simulink model "SimulationSimConnect"  (R2020b)
settings: Solver=FixedStepDiscrete  StartTime=0.0  StopTime=inf  RelTol=1e-3
InitFcn:
  | run('fbw_data_init_fbw_input.m')
values from neighbouring files (symbols this model uses):
  fbw_input_MATLABStruct = struct    [fbw_data_init_fbw_input.m]
undefined symbols (not defined in the file or in its folder): data, input, time
libraries: SimConnectToolbox x4, fbw_library x1, aerolibanimutils x1
settings Model: DataDictionary=fbw_data.sldd  Creator=Andreas  LastModifiedBy=Andreas
settings DebuggingCC: InheritedTsInSrcMsg=none

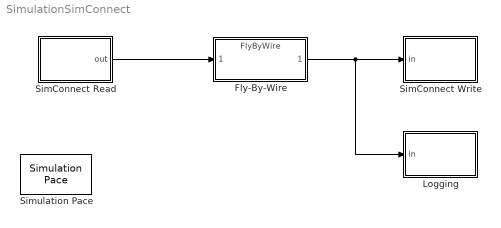
== system SimulationSimConnect ==
  Fly-By-Wire : ModelReference  ModelNameDialog=FlyByWire  ModelReferenceVersion=1.523
  Logging : Subsystem
  SimConnect Read : Subsystem
  SimConnect Write : Subsystem
  Simulation Pace : aerolibanimutils/Simulation Pace  SimulationPace=1  SleepMode=Auto  OutputPaceError=off  SampleTime=1/50
      settings: AttributesFormatString=%<SampleTime>
  wires:
  SimConnect Read/1(out) -> Fly-By-Wire/1
  Fly-By-Wire/1 -> Logging/1(in), SimConnect Write/1(in)

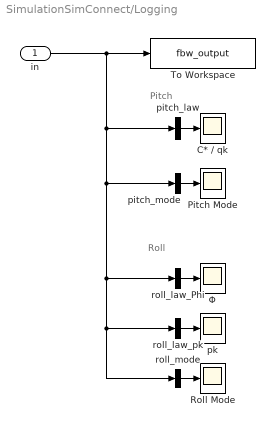
== system SimulationSimConnect/Logging ==
  note: Pitch
  note: Roll
  in : Inport
  C* / qk : Scope
  Pitch Mode : Scope
  Roll Mode : Scope
  To Workspace : ToWorkspace  VariableName=fbw_output  SaveFormat=Timeseries  SampleTime=-1
      settings: MaxDataPoints=30000
  pitch_law : BusSelector  OutputSignals=pitch.law_normal.nz_c_g,pitch.law_normal.Cstar_g,sim.data.nz_g,sim.data.qk_deg_s  OutputAsBus=on
  pitch_mode : BusSelector  OutputSignals=sim.data_computed.on_ground,pitch.data_computed.in_flight,pitch.data_computed.in_flare,pitch.data_computed.in_flight_gain  OutputAsBus=on
  pk : Scope
  roll_law_Phi : BusSelector  OutputSignals=roll.law_normal.Phi_c_deg,sim.data.Phi_deg  OutputAsBus=on
  roll_law_pk : BusSelector  OutputSignals=roll.law_normal.pk_c_deg_s,sim.data.pk_deg_s  OutputAsBus=on
  roll_mode : BusSelector  OutputSignals=sim.data_computed.on_ground,roll.data_computed.in_flight,roll.data_computed.in_flight_gain  OutputAsBus=on
  Φ : Scope
  wires:
  pitch_law/1 -> C* / qk/1
  roll_law_pk/1 -> pk/1
  roll_law_Phi/1 -> Φ/1
  in/1 -> To Workspace/1, pitch_law/1, roll_law_pk/1, roll_mode/1, roll_law_Phi/1, pitch_mode/1
  pitch_mode/1 -> Pitch Mode/1
  roll_mode/1 -> Roll Mode/1

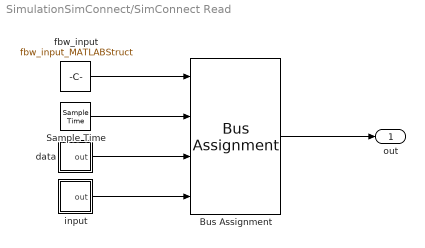
== system SimulationSimConnect/SimConnect Read ==
  Bus Assignment : BusAssignment  AssignedSignals=time.dt,data,input
  Sample Time : fbw_library/Sample Time  SystemSampleTime=-1  VariantActivationTime=update diagram  Latency=0  AutoFrameSizeCalculation=off
  data : Subsystem
  fbw_input : Constant  Value=fbw_input_MATLABStruct  OutDataTypeStr=Bus: fbw_input
  input : Subsystem
  out : Outport
  wires:
  fbw_input/1 -> Bus Assignment/1
  data/1(out) -> Bus Assignment/3
  Bus Assignment/1 -> out/1
  input/1(out) -> Bus Assignment/4
  Sample Time/1 -> Bus Assignment/2

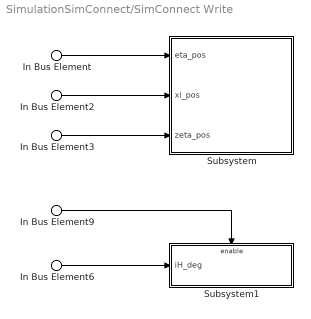
== system SimulationSimConnect/SimConnect Write ==
  In Bus Element : Inport  PortName=in  Element=sim.raw.output.eta_pos
  In Bus Element6 : Inport  PortName=in  Element=sim.raw.output.eta_trim_deg
  In Bus Element2 : Inport  PortName=in  Element=sim.raw.output.xi_pos
  In Bus Element3 : Inport  PortName=in  Element=sim.raw.output.zeta_pos
  In Bus Element9 : Inport  PortName=in  Element=sim.raw.output.eta_trim_deg_should_write
  Subsystem : Subsystem
  Subsystem1 : Subsystem
  wires:
  In Bus Element/1 -> Subsystem/1(eta_pos)
  In Bus Element2/1 -> Subsystem/2(xi_pos)
  In Bus Element3/1 -> Subsystem/3(zeta_pos)
  In Bus Element6/1 -> Subsystem1/1(iH_deg)
  In Bus Element9/1 -> Subsystem1/Enable

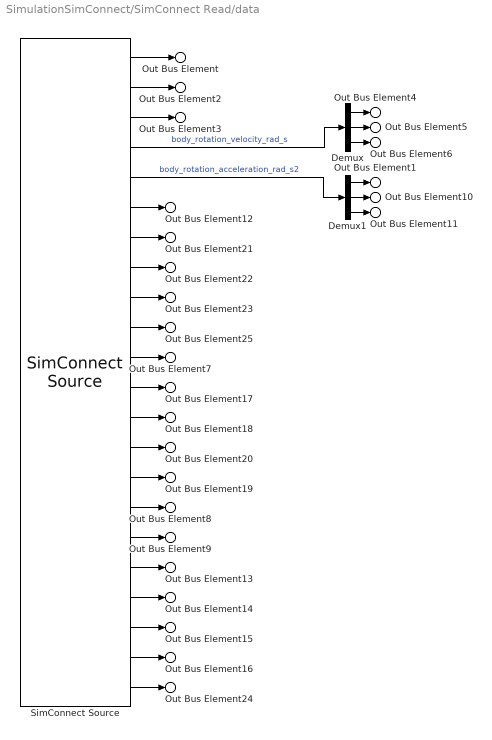
== system SimulationSimConnect/SimConnect Read/data ==
  Demux : Demux  Outputs=3
  Demux1 : Demux  Outputs=3
  SimConnect Source : SimConnectToolbox/SimConnect Source  configurationIndex=0  connectionName=SimConnectSource  variables=|
      | G FORCE, GFORCE;
      | PLANE PITCH DEGREES, DEGREE;
      | PLANE BANK DEGREES, DEGREE;
      | STRUCT BODY ROTATION VELOCITY, STRUCT;
      | STRUCT BODY ROTATION ACCELERATION, STRUCT;
      | ELEVATOR TRIM POSITION, DEGREE;
      | RUDDER TRIM PCT, PERCENT OVER 100;
      | INCIDENCE ALPHA, DEGREE;
      | INCIDENCE BETA, DEGREE;
      | BETA DOT, DEGREE PER SECOND;
      | AIRSPEED INDICATED, KNOTS;
      | AIRSPEED TRUE, KNOTS;
      | AIRSPEED MACH, MACH;
      | PLANE ALTITUDE, FEET;
      | INDICATED ALTITUDE, FEET;
      | RADIO HEIGHT, FEET;
      | CG PERCENT, PERCENT OVER 100;
      | GEAR ANIMATION POSITION:0, NUMBER;
      | GEAR ANIMATION POSITION:1, NUMBER;
      | GEAR ANIMATION POSITION:2, NUMBER;
      | FLAPS HANDLE INDEX, NUMBER;
      | AUTOPILOT MASTER, BOOL;
      settings: SourceProductName=SimConnect Toolbox
  Out Bus Element : Outport  PortName=out  Element=nz_g
  Out Bus Element2 : Outport  PortName=out  Element=Theta_deg
  Out Bus Element3 : Outport  PortName=out  Element=Phi_deg
  Out Bus Element4 : Outport  PortName=out  Element=q_rad_s
  Out Bus Element5 : Outport  PortName=out  Element=r_rad_s
  Out Bus Element6 : Outport  PortName=out  Element=p_rad_s
  Out Bus Element1 : Outport  PortName=out  Element=q_dot_rad_s2
  Out Bus Element10 : Outport  PortName=out  Element=r_dot_rad_s2
  Out Bus Element11 : Outport  PortName=out  Element=p_dot_rad_s2
  Out Bus Element12 : Outport  PortName=out  Element=eta_trim_deg
  Out Bus Element21 : Outport  PortName=out  Element=zeta_trim_pos
  Out Bus Element22 : Outport  PortName=out  Element=alpha_deg
  Out Bus Element23 : Outport  PortName=out  Element=beta_deg
  Out Bus Element25 : Outport  PortName=out  Element=beta_dot_deg_s
  Out Bus Element7 : Outport  PortName=out  Element=V_ias_kn
  Out Bus Element17 : Outport  PortName=out  Element=V_tas_kn
  Out Bus Element18 : Outport  PortName=out  Element=V_mach
  Out Bus Element20 : Outport  PortName=out  Element=H_ft
  Out Bus Element19 : Outport  PortName=out  Element=H_ind_ft
  Out Bus Element8 : Outport  PortName=out  Element=H_radio_ft
  Out Bus Element9 : Outport  PortName=out  Element=CG_percent_MAC
  Out Bus Element13 : Outport  PortName=out  Element=gear_animation_pos_0
  Out Bus Element14 : Outport  PortName=out  Element=gear_animation_pos_1
  Out Bus Element15 : Outport  PortName=out  Element=gear_animation_pos_2
  Out Bus Element16 : Outport  PortName=out  Element=flaps_handle_index
  Out Bus Element24 : Outport  PortName=out  Element=autopilot_master_on
  wires:
  Demux/3 -> Out Bus Element6/1
  SimConnect Source/3 -> Out Bus Element3/1
  SimConnect Source/4 -> Demux/1  "body_rotation_velocity_rad_s"
  Demux/2 -> Out Bus Element5/1
  SimConnect Source/1 -> Out Bus Element/1
  SimConnect Source/2 -> Out Bus Element2/1
  Demux/1 -> Out Bus Element4/1
  SimConnect Source/5 -> Demux1/1  "body_rotation_acceleration_rad_s2"
  Demux1/3 -> Out Bus Element11/1
  Demux1/1 -> Out Bus Element1/1
  Demux1/2 -> Out Bus Element10/1
  SimConnect Source/6 -> Out Bus Element12/1
  SimConnect Source/7 -> Out Bus Element21/1
  SimConnect Source/8 -> Out Bus Element22/1
  SimConnect Source/9 -> Out Bus Element23/1
  SimConnect Source/10 -> Out Bus Element25/1
  SimConnect Source/11 -> Out Bus Element7/1
  SimConnect Source/12 -> Out Bus Element17/1
  SimConnect Source/22 -> Out Bus Element24/1
  SimConnect Source/21 -> Out Bus Element16/1
  SimConnect Source/20 -> Out Bus Element15/1
  SimConnect Source/19 -> Out Bus Element14/1
  SimConnect Source/18 -> Out Bus Element13/1
  SimConnect Source/17 -> Out Bus Element9/1
  SimConnect Source/16 -> Out Bus Element8/1
  SimConnect Source/15 -> Out Bus Element19/1
  SimConnect Source/14 -> Out Bus Element20/1
  SimConnect Source/13 -> Out Bus Element18/1

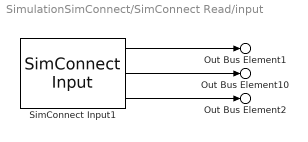
== system SimulationSimConnect/SimConnect Read/input ==
  SimConnect Input1 : SimConnectToolbox/SimConnect Input  configurationIndex=0  connectionName=SimConnectInput  variables=|
      | AXIS_ELEVATOR_SET, TRUE;
      | AXIS_AILERONS_SET, TRUE;
      | AXIS_RUDDER_SET, TRUE;
      settings: SourceProductName=SimConnect Toolbox
  Out Bus Element1 : Outport  PortName=out  Element=delta_eta_pos
  Out Bus Element10 : Outport  PortName=out  Element=delta_xi_pos
  Out Bus Element2 : Outport  PortName=out  Element=delta_zeta_pos
  wires:
  SimConnect Input1/1 -> Out Bus Element1/1
  SimConnect Input1/2 -> Out Bus Element10/1
  SimConnect Input1/3 -> Out Bus Element2/1

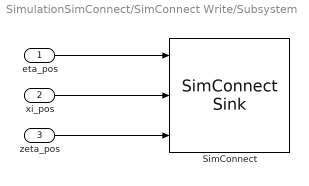
== system SimulationSimConnect/SimConnect Write/Subsystem ==
  eta_pos : Inport
  xi_pos : Inport  Port=2
  zeta_pos : Inport  Port=3
  SimConnect : SimConnectToolbox/SimConnect Sink  configurationIndex=0  connectionName=SimConnectSink  variables=|
      | ELEVATOR POSITION, POSITION;
      | AILERON POSITION, POSITION;
      | RUDDER POSITION, POSITION;
      settings: SourceProductName=SimConnect Toolbox
  wires:
  eta_pos/1 -> SimConnect/1
  xi_pos/1 -> SimConnect/2
  zeta_pos/1 -> SimConnect/3

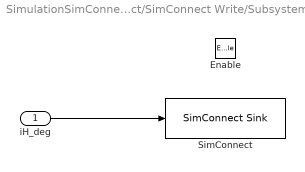
== system SimulationSimConnect/SimConnect Write/Subsystem1 ==
  iH_deg : Inport
  Enable : EnablePort
  SimConnect : SimConnectToolbox/SimConnect Sink  configurationIndex=0  connectionName=SimConnectSink  variables=ELEVATOR TRIM POSITION, DEGREE;
      settings: SourceProductName=SimConnect Toolbox
  wires:
  iH_deg/1 -> SimConnect/1
